simulink model "MDR_AA_TMD_Intercepteur"  (R2019b)
settings: Solver=ode4  StartTime=0.0  StopTime=Inf  FixedStep=0.01  RelTol=1e-3
values from neighbouring files (symbols this model uses):
  stdatm = [0 100 200 300 400 500 600 700 800 900 1000 1100 ... (4305 elements, 861x5)]    [stdatm.mat]
undefined symbols (not defined in the file or in its folder): Aero_Struct_CM, Aero_TMD, e0_0, e1_0, e2_0, e3_0, magnitude, Masse_Inertie_TMD, pow, Propu_TMD, Simu_TMD, Vm_0, xme_0
libraries: simulink x17
(part 2 of 4)

== system MDR_AA_TMD_Intercepteur/Intercepteur_TMD/Forces-Moments/Propulsion de l'exemple TMD ==
  <PS> : Inport
  Concaténation des deux phases de poussée : Subsystem
  Propulsion Booster : Subsystem  mask(Propulsion à poudre v1.0){Retard_Propu=Propu_TMD.Boost.Retard, t_b=Propu_TMD.Boost.Duree, Booster_Isp=Propu_TMD.Boost.ISP, Booster_Masse=Propu_TMD.Boost.Masse, Booster_Rapport=Propu_TMD.Boost.Profil, Diametre_tuy=Propu_TMD.Boost.D_Tuy, g0=9.80665}
      mask prompts: Retard_Propu "Retard Propulsion / T0 simu (s)"; t_b "Durée propulsion (s)"; Booster_Isp "Isp (s)"; Booster_Masse "Masse de poudre (kg)"; Booster_Rapport "Rapport de profil poussée (0->1)"; Diametre_tuy "Diamètre de la tuyere (m)"; g0 "Gravité au niveau du sol (m/s²)"
      mask help:
      | Modèle de propulseur à poudre.
      |
      | ENTREES
      | Pression_statique: Pression statique en Pa
      |
      | SORTIES
      | Force_poussee : Force de poussée axiale (en Newton)
      | débit_propu : Débit de combustible en kg.s^(-1)
      |
      | PARAMETRES
      | Retard Propulsion / T0 simu: délais entre le début de la simulation et l'allumage du propulseur
      | Durée propulsion: durée de la phase de propulsion (en s)
      | Isp: impulsion spécifique (en s)
      | Masse de poudre: Masse de propergol (en kg)
      | Rapport du profil de poussee (0->1): Allure du profil de poussée
      mask Help: eval('OpenHelp(''A3_NG.mdl'', ''Help\html\A3_NG_Model_Propu_Poudre_v10.html'')');
  Propulsion Croisiere : Subsystem  mask(Propulsion à poudre v1.0){Retard_Propu=Propu_TMD.Croisiere.Retard, t_b=Propu_TMD.Croisiere.Duree, Booster_Isp=Propu_TMD.Croisiere.ISP, Booster_Masse=Propu_TMD.Croisiere.Masse, Booster_Rapport=Propu_TMD.Croisiere.Profil, Diametre_tuy=Propu_TMD.Croisiere.D_Tuy, g0=9.80665}
      mask prompts: Retard_Propu "Retard Propulsion / T0 simu (s)"; t_b "Durée propulsion (s)"; Booster_Isp "Isp (s)"; Booster_Masse "Masse de poudre (kg)"; Booster_Rapport "Rapport de profil poussée (0->1)"; Diametre_tuy "Diamètre de la tuyere (m)"; g0 "Gravité au niveau du sol (m/s²)"
      mask help:
      | Modèle de propulseur à poudre.
      |
      | ENTREES
      | Pression_statique: Pression statique en Pa
      |
      | SORTIES
      | Force_poussee : Force de poussée axiale (en Newton)
      | débit_propu : Débit de combustible en kg.s^(-1)
      |
      | PARAMETRES
      | Retard Propulsion / T0 simu: délais entre le début de la simulation et l'allumage du propulseur
      | Durée propulsion: durée de la phase de propulsion (en s)
      | Isp: impulsion spécifique (en s)
      | Masse de poudre: Masse de propergol (en kg)
      | Rapport du profil de poussee (0->1): Allure du profil de poussée
      mask Help: eval('OpenHelp(''A3_NG.mdl'', ''Help\html\A3_NG_Model_Propu_Poudre_v10.html'')');
  Fpropu : Outport
  debit_carburant : Outport  Port=2
  wires:
  Concaténation des deux phases de poussée/2(debit_carburant) -> debit_carburant/1
  Propulsion Croisiere/2(debit_propu) -> Concaténation des deux phases de poussée/4(Debit_Croisiere)
  Propulsion Booster/1(Force_poussee) -> Concaténation des deux phases de poussée/1(Poussee_Boost)
  Propulsion Booster/2(debit_propu) -> Concaténation des deux phases de poussée/2(Poussee_Croisiere)
  Concaténation des deux phases de poussée/1(Fpropu) -> Fpropu/1
  <PS>/1 -> Propulsion Croisiere/1(Pression_statique), Propulsion Booster/1(Pression_statique)
  Propulsion Croisiere/1(Force_poussee) -> Concaténation des deux phases de poussée/3(Debit_Boost)

== system MDR_AA_TMD_Intercepteur/Modèle de terre/Modèle de terre WGS-84/Computation of Earth curvature radius (WGS-84) ==
  note: Computation of Earth curvature radius (WGS-84)
  Latitude : Inport
  1st Earth excentricity : Constant  Value=e
  Earth equatorial radius : Constant  Value=a
  Mux : Mux  Inputs=2
  Mux1 : Mux  Inputs=3
  Mux2 : Mux  Inputs=2
  Re = sqrt( Rmeridian * Rnormal ) : Fcn  Expr=sqrt(u(1)*u(2))
  "Rmeridian  = a ( 1 - e² ) / w^3 " : Fcn  Tag=Rmeridian  Expr=u(1)*(1-u(2)^2)/u(3)^3
  Rnormal = a / w : Fcn  Expr=u[1]/u[3]
  "w = sqrt ( 1 - e² sin² ( lat ) ) " : Fcn  Expr=sqrt(1-u(1)^2*sin(u(2))^2)
  Rmeridian : Outport  VectorParamsAs1DForOutWhenUnconnected=off
  Rnormal : Outport  Port=2  VectorParamsAs1DForOutWhenUnconnected=off
  Re : Outport  Port=3  VectorParamsAs1DForOutWhenUnconnected=off
  wires:
  "Rmeridian  = a ( 1 - e² ) / w^3 "/1 -> Rmeridian/1, Mux2/1
  Rnormal = a / w/1 -> Rnormal/1, Mux2/2
  Mux1/1 -> "Rmeridian  = a ( 1 - e² ) / w^3 "/1, Rnormal = a / w/1
  Earth equatorial radius/1 -> Mux1/1
  1st Earth excentricity/1 -> Mux/1, Mux1/2
  Latitude/1 -> Mux/2
  Re = sqrt( Rmeridian * Rnormal )/1 -> Re/1
  "w = sqrt ( 1 - e² sin² ( lat ) ) "/1 -> Mux1/3
  Mux/1 -> "w = sqrt ( 1 - e² sin² ( lat ) ) "/1
  Mux2/1 -> Re = sqrt( Rmeridian * Rnormal )/1

== system MDR_AA_TMD_Intercepteur/Modèle de terre/Modèle de terre WGS-84/Computation of the local gravity ==
  note: Computation of local gravity (WGS-84)
  Latitude : Inport
  Altitude : Inport  Port=2
  1st Earth excentricity : Constant  Value=e
  Earth equatorial radius : Constant  Value=a
  Ellipsoidal flattening : Constant  Value=f
  Gravity formula constant 1 : Constant  Value=k
  Gravity formula constant 2 : Constant  Value=m
  Mux : Mux  Inputs=6
  Mux1 : Mux
  Mux2 : Mux  Inputs=2
  Theoretical equatorial gravity : Constant  Value=ge
  g=ge*(1+k sin(lat)²)/w : Fcn  Expr=u(1)*(1+u(2)*sin(u(4))^2)/u(3)
  gh = g ( 1 - 2/a ( 1 + f + m - 2 f sin(lat)²) h + 3/a² h²) : Fcn  Expr=u[1]*(1-2/u[2]*(1+u[3]+u[4]-2*u[3]*sin(u[5])^2)*u[6]+3/u[2]^2*u[6]^2)
  "w = sqrt ( 1 - e² sin² ( lat ) ) " : Fcn  Expr=sqrt(1-u(1)^2*sin(u(2))^2)
  Gravity : Outport  VectorParamsAs1DForOutWhenUnconnected=off
  wires:
  Altitude/1 -> Mux/6
  Gravity formula constant 2/1 -> Mux/4
  Ellipsoidal flattening/1 -> Mux/3
  Earth equatorial radius/1 -> Mux/2
  g=ge*(1+k sin(lat)²)/w/1 -> Mux/1
  "w = sqrt ( 1 - e² sin² ( lat ) ) "/1 -> Mux1/3
  Mux2/1 -> "w = sqrt ( 1 - e² sin² ( lat ) ) "/1
  Latitude/1 -> Mux/5, Mux1/4, Mux2/2
  1st Earth excentricity/1 -> Mux2/1
  Mux/1 -> gh = g ( 1 - 2/a ( 1 + f + m - 2 f sin(lat)²) h + 3/a² h²)/1
  gh = g ( 1 - 2/a ( 1 + f + m - 2 f sin(lat)²) h + 3/a² h²)/1 -> Gravity/1
  Theoretical equatorial gravity/1 -> Mux1/1
  Gravity formula constant 1/1 -> Mux1/2
  Mux1/1 -> g=ge*(1+k sin(lat)²)/w/1

== system MDR_AA_TMD_Intercepteur/Modèle de terre/xyz_NED2LLA/ECEF2LLA ==
  ECEF : Inport
  Calcul de h : Subsystem
  Calcul de la latitude : Subsystem
  Calcul de la longitude : Subsystem
  Calcul de r : Subsystem
  Vector Concatenate1 : Concatenate  NumInputs=3
  LLA : Outport  VectorParamsAs1DForOutWhenUnconnected=off
  wires:
  ECEF/1 -> Calcul de r/1(xyz_ECEF), Calcul de h/3(xyz_ECEF), Calcul de la longitude/1(xyz_ECEF), Calcul de la latitude/1(xyz_ECEF)
  Calcul de h/1(h) -> Vector Concatenate1/3
  Vector Concatenate1/1 -> LLA/1
  Calcul de r/1(r) -> Calcul de la latitude/2(r), Calcul de h/2(r)
  Calcul de la longitude/1(Lambda) -> Vector Concatenate1/2
  Calcul de la latitude/1(Phi) -> Calcul de h/1(phi), Vector Concatenate1/1

== system MDR_AA_TMD_Intercepteur/Modèle de terre/xyz_NED2LLA/xyz_ENU2ECEF ==
  xyz_ENU : Inport
  Add : Sum
  Gain2 : Gain  Gain=[1;1;-1]
  Matrice de passage du repère NED au repère ECEF : Subsystem
  Product : Product  Multiplication=Matrix(*)
  Reshape : Reshape  OutputDimensionality=Column vector (2-D)
  Selector3 : Selector  InputPortWidth=3  IndexOptions=Index vector (dialog)  Indices=[2 1 3]  OutputSizes=1
  XYZ0 : Subsystem
  ECEF : Outport  VectorParamsAs1DForOutWhenUnconnected=off
  wires:
  xyz_ENU/1 -> Selector3/1
  Matrice de passage du repère NED au repère ECEF/1(M_NED2ECEF) -> Product/1
  XYZ0/1(XYZ0) -> Add/1
  Product/1 -> Add/2
  Add/1 -> ECEF/1
  Reshape/1 -> Product/2
  Gain2/1 -> Reshape/1
  Selector3/1 -> Gain2/1

== system MDR_AA_TMD_Intercepteur/Cible/Cible Cinématique v1.1/Actionneur Simulight/Retard Angle ==
  Angle_t_1 : Inport
  Angle_C : Inport  Port=2
  Tau : Inport  Port=3
  Constant1 : Constant
  Divide : Product  Inputs=*/
  Divide1 : Product  Inputs=**
  Gain : Gain  Gain=-1
  Gestion division par 0 : Subsystem
  Math Function : Math  SaturateOnIntegerOverflow=on
  Memory2 : Memory
  Ramp : simulink/Sources/Ramp  slope=1  start=0  InitialOutput=0
  Sum : Sum  Inputs=|-+
  Sum1 : Sum
  Sum2 : Sum  Inputs=-+
  Sum3 : Sum  Inputs=|+-
  Angle_R : Outport  VectorParamsAs1DForOutWhenUnconnected=off
  wires:
  Gestion division par 0/1(Non_zero) -> Divide/2
  Tau/1 -> Gestion division par 0/1(Zero_Possible)
  Angle_C/1 -> Sum2/2
  Divide1/1 -> Sum1/2
  Sum1/1 -> Angle_R/1
  Constant1/1 -> Sum/2
  Sum/1 -> Divide1/2
  Sum2/1 -> Divide1/1
  Math Function/1 -> Sum/1
  Gain/1 -> Divide/1
  Divide/1 -> Math Function/1
  Angle_t_1/1 -> Sum1/1, Sum2/1
  Ramp/1 -> Memory2/1, Sum3/1
  Memory2/1 -> Sum3/2
  Sum3/1 -> Gain/1

== system MDR_AA_TMD_Intercepteur/Cible/Cible Cinématique v1.1/Actionneur Simulight1/Retard Angle ==
  Angle_t_1 : Inport
  Angle_C : Inport  Port=2
  Tau : Inport  Port=3
  Constant1 : Constant
  Divide : Product  Inputs=*/
  Divide1 : Product  Inputs=**
  Gain : Gain  Gain=-1
  Gestion division par 0 : Subsystem
  Math Function : Math  SaturateOnIntegerOverflow=on
  Memory2 : Memory
  Ramp : simulink/Sources/Ramp  slope=1  start=0  InitialOutput=0
  Sum : Sum  Inputs=|-+
  Sum1 : Sum
  Sum2 : Sum  Inputs=-+
  Sum3 : Sum  Inputs=|+-
  Angle_R : Outport  VectorParamsAs1DForOutWhenUnconnected=off
  wires:
  Gestion division par 0/1(Non_zero) -> Divide/2
  Tau/1 -> Gestion division par 0/1(Zero_Possible)
  Angle_C/1 -> Sum2/2
  Divide1/1 -> Sum1/2
  Sum1/1 -> Angle_R/1
  Constant1/1 -> Sum/2
  Sum/1 -> Divide1/2
  Sum2/1 -> Divide1/1
  Math Function/1 -> Sum/1
  Gain/1 -> Divide/1
  Divide/1 -> Math Function/1
  Angle_t_1/1 -> Sum1/1, Sum2/1
  Ramp/1 -> Memory2/1, Sum3/1
  Memory2/1 -> Sum3/2
  Sum3/1 -> Gain/1

== system MDR_AA_TMD_Intercepteur/Cible/Cible Cinématique v1.1/Aero/Norme ==
  V : Inport
  Dot Product : DotProduct  InputSameDT=on  OutDataTypeStr=Inherit: Inherit via internal rule
  Sqrt : Math  Operator=sqrt  SaturateOnIntegerOverflow=on
  ||V|| : Outport  VectorParamsAs1DForOutWhenUnconnected=off
  wires:
  Sqrt/1 -> ||V||/1
  V/1 -> Dot Product/2, Dot Product/1
  Dot Product/1 -> Sqrt/1

== system MDR_AA_TMD_Intercepteur/Cible/Cible Cinématique v1.1/Aero/q\ ==
  ||V|| : Inport
  Rho : Inport  Port=2
  Gain : Gain  Gain=0.5
  Gain1 : Gain  Gain=(Lref^2*pi)/4
  Math Function : Math  Operator=magnitude^2  SaturateOnIntegerOverflow=on
  Product2 : Product  RndMeth=Zero
  rsv2 : Outport  VectorParamsAs1DForOutWhenUnconnected=off
  wires:
  Gain/1 -> Product2/1
  ||V||/1 -> Math Function/1
  Rho/1 -> Gain/1
  Product2/1 -> Gain1/1
  Math Function/1 -> Product2/2
  Gain1/1 -> rsv2/1

== system MDR_AA_TMD_Intercepteur/Cible/Cible Cinématique v1.1/Cinématique 6ddl Simulight avec pilotage en force/Calcul de la vitesse engin dans le repère inertiel ==
  Vb : Inport
  e0e1e2e3 : Inport  Port=2
  Math Function : Math  Operator=transpose  SaturateOnIntegerOverflow=on
  Product : Product  Multiplication=Matrix(*)  SaturateOnIntegerOverflow=on  InputSameDT=on  OutDataTypeStr=Inherit: Same as first input
  Quaternion2DCM : Subsystem  mask(Quaternion2DCM){}
      mask help:
      | Calcul la matrice de passage DCM (Direct Cosine Matrix) à partir du quaternion q.
      |
      | Si q = q0+ q1 i + q2 j + q3 k alors
      |
      | DCM = [
      | 1-2q2^2-2q3^2	2q1q2-2q0q3	2q1q3+2q0q2
      | 2q1q2+2q0q3	1-2q1^2-2q3^2	2q2q3-2q0q1
      | 2q1q3-2q0q2	2q2q3+2q0q1	1-2q1^2-2q2^2
      | ]
      mask Help: eval('OpenHelp(''A3_NG.mdl'', ''Help\html\A3_NG_Model_Quaternion2DCM.html'')');
  Ve : Outport  VectorParamsAs1DForOutWhenUnconnected=off
  wires:
  Vb/1 -> Product/2
  Math Function/1 -> Product/1
  e0e1e2e3/1 -> Quaternion2DCM/1(Quaternion)
  Quaternion2DCM/1(DCM) -> Math Function/1
  Product/1 -> Ve/1

== system MDR_AA_TMD_Intercepteur/Cible/Cible Cinématique v1.1/Cinématique 6ddl Simulight avec pilotage en force/Calcul des pqr ==
  Ab : Inport
  Vb : Inport  Port=2
  AlphaR : Inport  Port=3
  BetaR : Inport  Port=4
  pqr_force : Inport  Port=5
  Add : Sum  Inputs=+++
  pqr_a : Subsystem
  pqr_b : Subsystem
  pqr : Outport  VectorParamsAs1DForOutWhenUnconnected=off
  wires:
  AlphaR/1 -> pqr_a/1(AlphaR)
  BetaR/1 -> pqr_a/2(BetaR)
  pqr_a/1(pqr_a) -> Add/2
  pqr_b/1(pqr_b) -> Add/1
  Ab/1 -> pqr_b/1(Ab)
  Vb/1 -> pqr_b/2(Vb)
  Add/1 -> pqr/1
  pqr_force/1 -> Add/3

== system MDR_AA_TMD_Intercepteur/Cible/Cible Cinématique v1.1/Cinématique 6ddl Simulight avec pilotage en force/Equations des forces ==
  g : Inport
  Faero : Inport  Port=2
  Masse : Inport  Port=3
  pqr : Inport  Port=4
  Divide : Product  Inputs=*/
  Gestion de sortie de rampe : Subsystem
  "Sous contrainte de la rampe, effort uniquement sur l'axe longitudinal" : Subsystem
  Switch : Switch  Criteria=u2 ~= 0
  U^V : Subsystem  mask(Produit Vectoriel){}
      mask help: Calcul le produit vectoriel de deux vecteur 3x1.
      mask Help: eval('OpenHelp(''A3_NG.mdl'', ''Help\html\A3_NG_Model_ProdVect.html'')');
      mask Display: disp('Produit\nVectoriel')
  m3 : Constant  Value=Vb0
  sum : Sum  Inputs=|++  SaturateOnIntegerOverflow=on  InputSameDT=on  OutDataTypeStr=Inherit: Same as first input
  sum1 : Sum  SaturateOnIntegerOverflow=on  InputSameDT=on  OutDataTypeStr=Inherit: Same as first input
  ub vb wb : Integrator  InitialConditionSource=external  InitialCondition=Vm_0
  Vb : Outport  VectorParamsAs1DForOutWhenUnconnected=off
  Ab : Outport  Port=2  VectorParamsAs1DForOutWhenUnconnected=off
  wires:
  U^V/1(c(1) c(2) c(3)) -> sum/2
  m3/1 -> ub vb wb/2
  sum/1 -> ub vb wb/1
  ub vb wb/1 -> Vb/1, U^V/1(a(1) a(2) a(3))
  pqr/1 -> U^V/2(b(1) b(2) b(3))
  Faero/1 -> Divide/1
  Masse/1 -> Divide/2
  Divide/1 -> sum1/2, Gestion de sortie de rampe/1(Fm)
  g/1 -> sum1/1
  sum1/1 -> "Sous contrainte de la rampe, effort uniquement sur l'axe longitudinal"/1(F), Switch/1
  Switch/1 -> Ab/1, sum/1
  Gestion de sortie de rampe/1(Sortie_Rampe) -> Switch/2
  "Sous contrainte de la rampe, effort uniquement sur l'axe longitudinal"/1(Fx) -> Switch/3

== system MDR_AA_TMD_Intercepteur/Cible/Cible Cinématique v1.1/Cinématique 6ddl Simulight avec pilotage en force/Intégration de la vitesse dans le repère inertiel ==
  Ve : Inport
  m2 : Constant  Value=Xe0
  xe ye ze : Integrator  InitialConditionSource=external  InitialCondition=xme_0
  Xe : Outport  VectorParamsAs1DForOutWhenUnconnected=off
  wires:
  m2/1 -> xe ye ze/2
  Ve/1 -> xe ye ze/1
  xe ye ze/1 -> Xe/1

== system MDR_AA_TMD_Intercepteur/Cible/Cible Cinématique v1.1/Cinématique 6ddl Simulight avec pilotage en force/Pesanteur ==
  Euler : Inport
  g : Inport  Port=2
  Gain : Gain  Gain=[0;0;1]
  Inert2Miss : Subsystem  mask(Inert2Miss){}
      mask help: Calcul les composantes d'un vecteur du repère inertiel dans le repère missile.
      mask Help: eval('OpenHelp(''A3_NG.mdl'', ''Help\html\A3_NG_Model_Inert2Miss.html'')');
  g_miss : Outport  VectorParamsAs1DForOutWhenUnconnected=off
  wires:
  Euler/1 -> Inert2Miss/1(Euler)
  g/1 -> Gain/1
  Gain/1 -> Inert2Miss/2(U)
  Inert2Miss/1(V) -> g_miss/1

== system MDR_AA_TMD_Intercepteur/Cible/Cible Cinématique v1.1/Cinématique 6ddl Simulight avec pilotage en force/Quaternion2Euler ==
  Quaternion : Inport  PortDimensions=[4 1]
  Fcn1 : Fcn  Expr=atan2( 2*(u(1)*u(2)+u(3)*u(4)),u(1)^2-u(2)^2-u(3)^2+u(4)^2 )
  Fcn3 : Fcn  Expr=atan2( 2*(u(2)*u(3)+u(1)*u(4)),u(1)^2+u(2)^2-u(3)^2-u(4)^2 )
  Fcn4 : Fcn  Expr=2*(u(1)*u(3)-u(2)*u(4))
  Fcn5 : Fcn  Expr=asin(u(1))
  Mux : Mux  Inputs=3
  Saturation : Saturate  UpperLimit=1  LowerLimit=-1
  Euler : Outport  VectorParamsAs1DForOutWhenUnconnected=off
  wires:
  Fcn5/1 -> Mux/2
  Saturation/1 -> Fcn5/1
  Fcn4/1 -> Saturation/1
  Quaternion/1 -> Fcn1/1, Fcn4/1, Fcn3/1
  Fcn3/1 -> Mux/3
  Mux/1 -> Euler/1
  Fcn1/1 -> Mux/1

== system MDR_AA_TMD_Intercepteur/Cible/Cible Cinématique v1.1/Cinématique 6ddl Simulight avec pilotage en force/pqr2Quaternion ==
  pqr : Inport
  Constant1 : Constant  Value=Euler_Init
  Divide : Product  Inputs=*/
  Euler2Quaternion : Subsystem  mask(Euler2Quaternion){}
      mask help:
      | Calcul du quaternion q à partir des angles d'Euler (phi,theta,psi)
      |
      | q = q0 + q1 i + q2 j + q3 k
      | avec :
      |
      | q0 = cos(0.5*psi)cos(0.5*theta)cos(0.5*phi) + sin(0.5*psi)sin(0.5*theta)sin(0.5*phi)
      | q1 =  sin(0.5*psi)cos(0.5*theta)cos(0.5*phi) - cos(0.5*psi)sin(0.5*theta)sin(0.5*phi)
      | q2 =  cos(0.5*psi)sin(0.5*theta)cos(0.5*phi) + sin(0.5*psi)cos(0.5*theta)sin(0.5*phi)
      | q3 =  cos(0.5*psi)cos(0.5*theta)sin(0.5*phi) - sin(0.5*psi)sin(0.5*theta)cos(0.5*phi)
      mask Help: eval('OpenHelp(''A3_NG.mdl'', ''Help\html\A3_NG_Model_Euler2Quaternion.html'')');
  Norme : Subsystem  mask(Norme){}
      mask help: Calcul la norme quadratique d'un vecteur.
      mask Help: eval('OpenHelp(''A3_NG.mdl'', ''Help\html\A3_NG_Model_Norme.html'')');
  deg2rad : Gain  Gain=pi/180
  e0 e1 e2 e3 : Integrator  InitialConditionSource=external  InitialCondition=[e0_0 e1_0 e2_0 e3_0]
  pqr to eidot : Subsystem
  Quaternion : Outport  VectorParamsAs1DForOutWhenUnconnected=off
  wires:
  deg2rad/1 -> Euler2Quaternion/1(Euler)
  pqr/1 -> pqr to eidot/1(pqr)
  Divide/1 -> Quaternion/1, pqr to eidot/2(e0e1e2e3)
  Norme/1(||V||) -> Divide/2
  e0 e1 e2 e3/1 -> Divide/1, Norme/1(V)
  Constant1/1 -> deg2rad/1
  pqr to eidot/1(eidot) -> e0 e1 e2 e3/1
  Euler2Quaternion/1(Quaternion) -> e0 e1 e2 e3/2

== system MDR_AA_TMD_Intercepteur/Cible/Cible Cinématique v1.1/Pilote 2 axes Simulight à partir de gradient/Alpha commandé - Plan de tangage ==
  GcoV : Inport
  Masse : Inport  Port=2
  Pression_dynamique : Inport  Port=3
  Compare To Zero : simulink/Logic and Bit Operations/Compare To Zero  relop===  OutDataTypeStr=boolean  ZeroCross=off
  Cza : Gain  Gain=Cza
  Divide1 : Product  Inputs=*/
  Memory : Memory
  Product : Product  RndMeth=Zero
  Switch : Switch  Criteria=u2 > Threshold
  Zero Offset : Subsystem  mask(Zero offset){tol=10^-6}
      mask prompts: tol "Tolerance"
      mask help: This block outputs a value equal to the tolerance specified in the block parameters if the input falls within a sphere with this tolerance as radius and center in the origin. Otherwise, the output equals the input.
      mask Help: eval('OpenHelp(''A3_Blockset.mdl'', ''..\Help\Toolbox\Tools\Zero_offset.html'')');
  Alphaco : Outport  PortDimensions=1  VectorParamsAs1DForOutWhenUnconnected=off
  wires:
  Cza/1 -> Compare To Zero/1, Zero Offset/1(In)
  Zero Offset/1(Out) -> Divide1/2
  Memory/1 -> Switch/1
  Product/1 -> Switch/3
  Divide1/1 -> Product/1
  Masse/1 -> Divide1/1
  GcoV/1 -> Product/2
  Compare To Zero/1 -> Switch/2
  Switch/1 -> Alphaco/1, Memory/1
  Pression_dynamique/1 -> Cza/1

== system MDR_AA_TMD_Intercepteur/Cible/Cible Cinématique v1.1/Pilote 2 axes Simulight à partir de gradient/Beta commandé - Plan de lacet ==
  GcoH : Inport
  Masse : Inport  Port=2
  Pression_dynamique : Inport  Port=3
  Compare To Zero : simulink/Logic and Bit Operations/Compare To Zero  relop===  OutDataTypeStr=boolean  ZeroCross=off
  Cyb : Gain  Gain=Cyb
  Divide1 : Product  Inputs=*/
  Memory : Memory
  Product : Product  RndMeth=Zero
  Switch : Switch  Criteria=u2 > Threshold
  Zero Offset : Subsystem  mask(Zero offset){tol=10^-6}
      mask prompts: tol "Tolerance"
      mask help: This block outputs a value equal to the tolerance specified in the block parameters if the input falls within a sphere with this tolerance as radius and center in the origin. Otherwise, the output equals the input.
      mask Help: eval('OpenHelp(''A3_Blockset.mdl'', ''..\Help\Toolbox\Tools\Zero_offset.html'')');
  Betaco : Outport  PortDimensions=1  VectorParamsAs1DForOutWhenUnconnected=off
  wires:
  Pression_dynamique/1 -> Cyb/1
  Switch/1 -> Memory/1, Betaco/1
  Compare To Zero/1 -> Switch/2
  GcoH/1 -> Product/2
  Masse/1 -> Divide1/1
  Divide1/1 -> Product/1
  Product/1 -> Switch/3
  Memory/1 -> Switch/1
  Zero Offset/1(Out) -> Divide1/2
  Cyb/1 -> Zero Offset/1(In), Compare To Zero/1

== system MDR_AA_TMD_Intercepteur/Cible/Cible Cinématique v1.1/Pilote 2 axes Simulight à partir de gradient/Norme ==
  V : Inport
  Dot Product : DotProduct  InputSameDT=on  OutDataTypeStr=Inherit: Inherit via internal rule
  Sqrt : Math  Operator=sqrt  SaturateOnIntegerOverflow=on
  ||V|| : Outport  VectorParamsAs1DForOutWhenUnconnected=off
  wires:
  Sqrt/1 -> ||V||/1
  V/1 -> Dot Product/2, Dot Product/1
  Dot Product/1 -> Sqrt/1

== system MDR_AA_TMD_Intercepteur/Cible/Cible Cinématique v1.1/Pilote 2 axes Simulight à partir de gradient/q\ ==
  ||V|| : Inport
  Rho : Inport  Port=2
  Gain : Gain  Gain=0.5
  Gain1 : Gain  Gain=(Lref^2*pi)/4
  Math Function : Math  Operator=magnitude^2  SaturateOnIntegerOverflow=on
  Product2 : Product  RndMeth=Zero
  rsv2 : Outport  VectorParamsAs1DForOutWhenUnconnected=off
  wires:
  Gain/1 -> Product2/1
  ||V||/1 -> Math Function/1
  Rho/1 -> Gain/1
  Product2/1 -> Gain1/1
  Math Function/1 -> Product2/2
  Gain1/1 -> rsv2/1

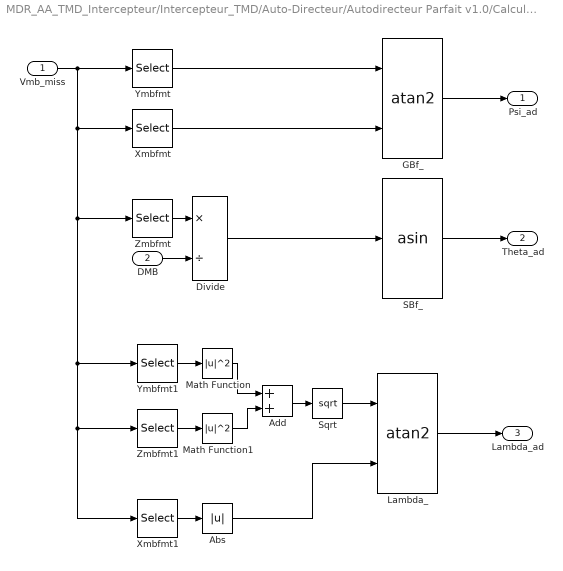
== system MDR_AA_TMD_Intercepteur/Intercepteur_TMD/Auto-Directeur/Autodirecteur Parfait v1.0/Calcul des angles site et gisement de la droite missile//but dans le repère missile ==
  Vmb_miss : Inport
  DMB : Inport  Port=2
  Abs : Abs
  Add : Sum
  Divide : Product  Inputs=*/
  GBf_ : Trigonometry  Operator=atan2
  Lambda_ : Trigonometry  Operator=atan2
  Math Function : Math  Operator=magnitude^2  SaturateOnIntegerOverflow=on
  Math Function1 : Math  Operator=magnitude^2  SaturateOnIntegerOverflow=on
  SBf_ : Trigonometry  Operator=asin
  Sqrt : Sqrt  SaturateOnIntegerOverflow=on
  Xmbfmt : Selector  InputPortWidth=3  IndexOptions=Index vector (dialog)  Indices=[1]  OutputSizes=1
  Xmbfmt1 : Selector  InputPortWidth=3  IndexOptions=Index vector (dialog)  Indices=[1]  OutputSizes=1
  Ymbfmt : Selector  InputPortWidth=3  IndexOptions=Index vector (dialog)  Indices=[2]  OutputSizes=1
  Ymbfmt1 : Selector  InputPortWidth=3  IndexOptions=Index vector (dialog)  Indices=[2]  OutputSizes=1
  Zmbfmt : Selector  InputPortWidth=3  IndexOptions=Index vector (dialog)  Indices=[3]  OutputSizes=1
  Zmbfmt1 : Selector  InputPortWidth=3  IndexOptions=Index vector (dialog)  Indices=[3]  OutputSizes=1
  Psi_ad : Outport  VectorParamsAs1DForOutWhenUnconnected=off
  Theta_ad : Outport  Port=2  VectorParamsAs1DForOutWhenUnconnected=off
  Lambda_ad : Outport  Port=3  VectorParamsAs1DForOutWhenUnconnected=off
  wires:
  DMB/1 -> Divide/2
  Divide/1 -> SBf_/1
  Zmbfmt/1 -> Divide/1
  SBf_/1 -> Theta_ad/1
  GBf_/1 -> Psi_ad/1
  Xmbfmt/1 -> GBf_/2
  Ymbfmt/1 -> GBf_/1
  Vmb_miss/1 -> Ymbfmt/1, Xmbfmt/1, Zmbfmt/1, Ymbfmt1/1, Zmbfmt1/1, Xmbfmt1/1
  Add/1 -> Sqrt/1
  Ymbfmt1/1 -> Math Function/1
  Math Function/1 -> Add/1
  Zmbfmt1/1 -> Math Function1/1
  Math Function1/1 -> Add/2
  Sqrt/1 -> Lambda_/1
  Xmbfmt1/1 -> Abs/1
  Abs/1 -> Lambda_/2
  Lambda_/1 -> Lambda_ad/1

== system MDR_AA_TMD_Intercepteur/Intercepteur_TMD/Auto-Directeur/Autodirecteur Parfait v1.0/Calcul des vitesses de défilements de la droite missile//but dans le repère missile ==
  Omega_miss : Inport
  Gain : Gain  Gain=-1
  omega ymt : Selector  InputPortWidth=3  IndexOptions=Index vector (dialog)  Indices=[2]  OutputSizes=1
  omega zmt : Selector  InputPortWidth=3  IndexOptions=Index vector (dialog)  Indices=[3]  OutputSizes=1
  wzad : Outport  VectorParamsAs1DForOutWhenUnconnected=off
  wyad : Outport  Port=2  VectorParamsAs1DForOutWhenUnconnected=off
  wires:
  omega zmt/1 -> wyad/1
  omega ymt/1 -> Gain/1
  Omega_miss/1 -> omega ymt/1, omega zmt/1
  Gain/1 -> wzad/1

== system MDR_AA_TMD_Intercepteur/Intercepteur_TMD/Auto-Directeur/Autodirecteur Parfait v1.0/Calcul du vecteur rotation instantané de la droite missile//but dans le repère inertiel ==
  Pos_Miss_inert : Inport
  Pos_Cible_inert : Inport  Port=2
  Vit_Miss_inert : Inport  Port=3
  Vit_Cible_inert : Inport  Port=4
  Add : Sum  Inputs=+-
  Add1 : Sum  Inputs=+-
  Divide : Product  Inputs=*/
  Math Function1 : Math  Operator=magnitude^2  SaturateOnIntegerOverflow=on
  Norme : Subsystem  mask(Norme){}
      mask help: Calcul la norme quadratique d'un vecteur.
      mask Help: eval('OpenHelp(''A3_NG.mdl'', ''Help\html\A3_NG_Model_Norme.html'')');
  U^V : Subsystem  mask(Produit Vectoriel){}
      mask help: Calcul le produit vectoriel de deux vecteur 3x1.
      mask Help: eval('OpenHelp(''A3_NG.mdl'', ''Help\html\A3_NG_Model_ProdVect.html'')');
      mask Display: disp('Produit\nVectoriel')
  Omega_inert : Outport  VectorParamsAs1DForOutWhenUnconnected=off
  wires:
  Divide/1 -> Omega_inert/1  "NPi"
  Norme/1(||V||) -> Math Function1/1
  Pos_Cible_inert/1 -> Add/1
  Pos_Miss_inert/1 -> Add/2
  Add/1 -> U^V/1(a(1) a(2) a(3)), Norme/1(V)  "dX"
  Vit_Miss_inert/1 -> Add1/2
  Vit_Cible_inert/1 -> Add1/1
  Add1/1 -> U^V/2(b(1) b(2) b(3))  "dV"
  U^V/1(c(1) c(2) c(3)) -> Divide/1
  Math Function1/1 -> Divide/2

== system MDR_AA_TMD_Intercepteur/Intercepteur_TMD/Auto-Directeur/Autodirecteur Parfait v1.0/Changement de repère inertiel -> miss ==
  Euler : Inport
  Omega_inert : Inport  Port=2
  Vmb_inert : Inport  Port=3
  Inert2Miss1 : Subsystem  mask(Inert2Miss){}
      mask help: Calcul les composantes d'un vecteur du repère inertiel dans le repère missile.
      mask Help: eval('OpenHelp(''A3_NG.mdl'', ''Help\html\A3_NG_Model_Inert2Miss.html'')');
  Matrix Concatenate : Concatenate  Mode=Multidimensional array  ConcatenateDimension=2
  Selector : Selector  NumberOfDimensions=2  InputPortWidth=[3 2]  IndexOptions=Select all,Index vector (dialog)  Indices=[1],1  OutputSizes=1,1
  Selector1 : Selector  NumberOfDimensions=2  InputPortWidth=[3 2]  IndexOptions=Select all,Index vector (dialog)  Indices=[1 3],2  OutputSizes=1,1
  Omega_miss : Outport  VectorParamsAs1DForOutWhenUnconnected=off
  Vmb_miss : Outport  Port=2  VectorParamsAs1DForOutWhenUnconnected=off
  wires:
  Euler/1 -> Inert2Miss1/1(Euler)
  Omega_inert/1 -> Matrix Concatenate/1
  Vmb_inert/1 -> Matrix Concatenate/2
  Matrix Concatenate/1 -> Inert2Miss1/2(U)
  Inert2Miss1/1(V) -> Selector/1, Selector1/1
  Selector/1 -> Omega_miss/1
  Selector1/1 -> Vmb_miss/1

== system MDR_AA_TMD_Intercepteur/Intercepteur_TMD/Auto-Directeur/Autodirecteur Parfait v1.0/Site et Gisement de la droite missile//but dans le repère inertiel ==
  Pos_Cible_inert : Inport
  Pos_Miss_inert : Inport  Port=2
  Add : Sum  Inputs=+-
  Norme : Subsystem  mask(Norme){}
      mask help: Calcul la norme quadratique d'un vecteur.
      mask Help: eval('OpenHelp(''A3_NG.mdl'', ''Help\html\A3_NG_Model_Norme.html'')');
  Vector Concatenate : Concatenate  NumInputs=3
  Xb : Selector  InputPortWidth=3  IndexOptions=Index vector (dialog)  Indices=[1]  OutputSizes=1
  Xb-Xm : Sum  Inputs=+-
  Xb-Xm1 : Sum  Inputs=+-
  Xm : Selector  InputPortWidth=3  IndexOptions=Index vector (dialog)  Indices=[1]  OutputSizes=1
  Yb : Selector  InputPortWidth=3  IndexOptions=Index vector (dialog)  Indices=[2]  OutputSizes=1
  Yb-Ym : Sum  Inputs=+-
  Ym : Selector  InputPortWidth=3  IndexOptions=Index vector (dialog)  Indices=[2]  OutputSizes=1
  Zb : Selector  InputPortWidth=3  IndexOptions=Index vector (dialog)  Indices=[3]  OutputSizes=1
  Zm : Selector  InputPortWidth=3  IndexOptions=Index vector (dialog)  Indices=[3]  OutputSizes=1
  Vmb_inert : Outport  VectorParamsAs1DForOutWhenUnconnected=off
  DMB : Outport  Port=2  VectorParamsAs1DForOutWhenUnconnected=off
  wires:
  Yb/1 -> Yb-Ym/1
  Ym/1 -> Yb-Ym/2
  Xb/1 -> Xb-Xm/1
  Xm/1 -> Xb-Xm/2
  Zb/1 -> Xb-Xm1/1
  Zm/1 -> Xb-Xm1/2
  Pos_Cible_inert/1 -> Zb/1, Add/1, Yb/1, Xb/1
  Pos_Miss_inert/1 -> Zm/1, Add/2, Ym/1, Xm/1
  Norme/1(||V||) -> DMB/1
  Add/1 -> Norme/1(V)
  Vector Concatenate/1 -> Vmb_inert/1
  Xb-Xm/1 -> Vector Concatenate/1
  Yb-Ym/1 -> Vector Concatenate/2
  Xb-Xm1/1 -> Vector Concatenate/3

== system MDR_AA_TMD_Intercepteur/Intercepteur_TMD/Bloc Cinématique/Cinématique 6ddl Simulight avec pilotage en force/Calcul de la vitesse engin dans le repère inertiel ==
  Vb : Inport
  e0e1e2e3 : Inport  Port=2
  Math Function : Math  Operator=transpose  SaturateOnIntegerOverflow=on
  Product : Product  Multiplication=Matrix(*)  SaturateOnIntegerOverflow=on  InputSameDT=on  OutDataTypeStr=Inherit: Same as first input
  Quaternion2DCM : Subsystem  mask(Quaternion2DCM){}
      mask help:
      | Calcul la matrice de passage DCM (Direct Cosine Matrix) à partir du quaternion q.
      |
      | Si q = q0+ q1 i + q2 j + q3 k alors
      |
      | DCM = [
      | 1-2q2^2-2q3^2	2q1q2-2q0q3	2q1q3+2q0q2
      | 2q1q2+2q0q3	1-2q1^2-2q3^2	2q2q3-2q0q1
      | 2q1q3-2q0q2	2q2q3+2q0q1	1-2q1^2-2q2^2
      | ]
      mask Help: eval('OpenHelp(''A3_NG.mdl'', ''Help\html\A3_NG_Model_Quaternion2DCM.html'')');
  Ve : Outport  VectorParamsAs1DForOutWhenUnconnected=off
  wires:
  Vb/1 -> Product/2
  Math Function/1 -> Product/1
  e0e1e2e3/1 -> Quaternion2DCM/1(Quaternion)
  Quaternion2DCM/1(DCM) -> Math Function/1
  Product/1 -> Ve/1

== system MDR_AA_TMD_Intercepteur/Intercepteur_TMD/Bloc Cinématique/Cinématique 6ddl Simulight avec pilotage en force/Calcul des pqr ==
  Ab : Inport
  Vb : Inport  Port=2
  AlphaR : Inport  Port=3
  BetaR : Inport  Port=4
  pqr_force : Inport  Port=5
  Add : Sum  Inputs=+++
  pqr_a : Subsystem
  pqr_b : Subsystem
  pqr : Outport  VectorParamsAs1DForOutWhenUnconnected=off
  wires:
  AlphaR/1 -> pqr_a/1(AlphaR)
  BetaR/1 -> pqr_a/2(BetaR)
  pqr_a/1(pqr_a) -> Add/2
  pqr_b/1(pqr_b) -> Add/1
  Ab/1 -> pqr_b/1(Ab)
  Vb/1 -> pqr_b/2(Vb)
  Add/1 -> pqr/1
  pqr_force/1 -> Add/3

== system MDR_AA_TMD_Intercepteur/Intercepteur_TMD/Bloc Cinématique/Cinématique 6ddl Simulight avec pilotage en force/Equations des forces ==
  g : Inport
  Faero : Inport  Port=2
  Masse : Inport  Port=3
  pqr : Inport  Port=4
  Divide : Product  Inputs=*/
  Gestion de sortie de rampe : Subsystem
  "Sous contrainte de la rampe, effort uniquement sur l'axe longitudinal" : Subsystem
  Switch : Switch  Criteria=u2 ~= 0
  U^V : Subsystem  mask(Produit Vectoriel){}
      mask help: Calcul le produit vectoriel de deux vecteur 3x1.
      mask Help: eval('OpenHelp(''A3_NG.mdl'', ''Help\html\A3_NG_Model_ProdVect.html'')');
      mask Display: disp('Produit\nVectoriel')
  m3 : Constant  Value=Vb0
  sum : Sum  Inputs=|++  SaturateOnIntegerOverflow=on  InputSameDT=on  OutDataTypeStr=Inherit: Same as first input
  sum1 : Sum  SaturateOnIntegerOverflow=on  InputSameDT=on  OutDataTypeStr=Inherit: Same as first input
  ub vb wb : Integrator  InitialConditionSource=external  InitialCondition=Vm_0
  Vb : Outport  VectorParamsAs1DForOutWhenUnconnected=off
  Ab : Outport  Port=2  VectorParamsAs1DForOutWhenUnconnected=off
  wires:
  U^V/1(c(1) c(2) c(3)) -> sum/2
  m3/1 -> ub vb wb/2
  sum/1 -> ub vb wb/1
  ub vb wb/1 -> Vb/1, U^V/1(a(1) a(2) a(3))
  pqr/1 -> U^V/2(b(1) b(2) b(3))
  Faero/1 -> Divide/1
  Masse/1 -> Divide/2
  Divide/1 -> sum1/2, Gestion de sortie de rampe/1(Fm)
  g/1 -> sum1/1
  sum1/1 -> "Sous contrainte de la rampe, effort uniquement sur l'axe longitudinal"/1(F), Switch/1
  Switch/1 -> Ab/1, sum/1
  Gestion de sortie de rampe/1(Sortie_Rampe) -> Switch/2
  "Sous contrainte de la rampe, effort uniquement sur l'axe longitudinal"/1(Fx) -> Switch/3

== system MDR_AA_TMD_Intercepteur/Intercepteur_TMD/Bloc Cinématique/Cinématique 6ddl Simulight avec pilotage en force/Intégration de la vitesse dans le repère inertiel ==
  Ve : Inport
  m2 : Constant  Value=Xe0
  xe ye ze : Integrator  InitialConditionSource=external  InitialCondition=xme_0
  Xe : Outport  VectorParamsAs1DForOutWhenUnconnected=off
  wires:
  m2/1 -> xe ye ze/2
  Ve/1 -> xe ye ze/1
  xe ye ze/1 -> Xe/1

== system MDR_AA_TMD_Intercepteur/Intercepteur_TMD/Bloc Cinématique/Cinématique 6ddl Simulight avec pilotage en force/Pesanteur ==
  Euler : Inport
  g : Inport  Port=2
  Gain : Gain  Gain=[0;0;1]
  Inert2Miss : Subsystem  mask(Inert2Miss){}
      mask help: Calcul les composantes d'un vecteur du repère inertiel dans le repère missile.
      mask Help: eval('OpenHelp(''A3_NG.mdl'', ''Help\html\A3_NG_Model_Inert2Miss.html'')');
  g_miss : Outport  VectorParamsAs1DForOutWhenUnconnected=off
  wires:
  Euler/1 -> Inert2Miss/1(Euler)
  g/1 -> Gain/1
  Gain/1 -> Inert2Miss/2(U)
  Inert2Miss/1(V) -> g_miss/1

== system MDR_AA_TMD_Intercepteur/Intercepteur_TMD/Bloc Cinématique/Cinématique 6ddl Simulight avec pilotage en force/Quaternion2Euler ==
  Quaternion : Inport  PortDimensions=[4 1]
  Fcn1 : Fcn  Expr=atan2( 2*(u(1)*u(2)+u(3)*u(4)),u(1)^2-u(2)^2-u(3)^2+u(4)^2 )
  Fcn3 : Fcn  Expr=atan2( 2*(u(2)*u(3)+u(1)*u(4)),u(1)^2+u(2)^2-u(3)^2-u(4)^2 )
  Fcn4 : Fcn  Expr=2*(u(1)*u(3)-u(2)*u(4))
  Fcn5 : Fcn  Expr=asin(u(1))
  Mux : Mux  Inputs=3
  Saturation : Saturate  UpperLimit=1  LowerLimit=-1
  Euler : Outport  VectorParamsAs1DForOutWhenUnconnected=off
  wires:
  Fcn5/1 -> Mux/2
  Saturation/1 -> Fcn5/1
  Fcn4/1 -> Saturation/1
  Quaternion/1 -> Fcn1/1, Fcn4/1, Fcn3/1
  Fcn3/1 -> Mux/3
  Mux/1 -> Euler/1
  Fcn1/1 -> Mux/1

== system MDR_AA_TMD_Intercepteur/Intercepteur_TMD/Bloc Cinématique/Cinématique 6ddl Simulight avec pilotage en force/pqr2Quaternion ==
  pqr : Inport
  Constant1 : Constant  Value=Euler_Init
  Divide : Product  Inputs=*/
  Euler2Quaternion : Subsystem  mask(Euler2Quaternion){}
      mask help:
      | Calcul du quaternion q à partir des angles d'Euler (phi,theta,psi)
      |
      | q = q0 + q1 i + q2 j + q3 k
      | avec :
      |
      | q0 = cos(0.5*psi)cos(0.5*theta)cos(0.5*phi) + sin(0.5*psi)sin(0.5*theta)sin(0.5*phi)
      | q1 =  sin(0.5*psi)cos(0.5*theta)cos(0.5*phi) - cos(0.5*psi)sin(0.5*theta)sin(0.5*phi)
      | q2 =  cos(0.5*psi)sin(0.5*theta)cos(0.5*phi) + sin(0.5*psi)cos(0.5*theta)sin(0.5*phi)
      | q3 =  cos(0.5*psi)cos(0.5*theta)sin(0.5*phi) - sin(0.5*psi)sin(0.5*theta)cos(0.5*phi)
      mask Help: eval('OpenHelp(''A3_NG.mdl'', ''Help\html\A3_NG_Model_Euler2Quaternion.html'')');
  Norme : Subsystem  mask(Norme){}
      mask help: Calcul la norme quadratique d'un vecteur.
      mask Help: eval('OpenHelp(''A3_NG.mdl'', ''Help\html\A3_NG_Model_Norme.html'')');
  deg2rad : Gain  Gain=pi/180
  e0 e1 e2 e3 : Integrator  InitialConditionSource=external  InitialCondition=[e0_0 e1_0 e2_0 e3_0]
  pqr to eidot : Subsystem
  Quaternion : Outport  VectorParamsAs1DForOutWhenUnconnected=off
  wires:
  deg2rad/1 -> Euler2Quaternion/1(Euler)
  pqr/1 -> pqr to eidot/1(pqr)
  Divide/1 -> Quaternion/1, pqr to eidot/2(e0e1e2e3)
  Norme/1(||V||) -> Divide/2
  e0 e1 e2 e3/1 -> Divide/1, Norme/1(V)
  Constant1/1 -> deg2rad/1
  pqr to eidot/1(eidot) -> e0 e1 e2 e3/1
  Euler2Quaternion/1(Quaternion) -> e0 e1 e2 e3/2

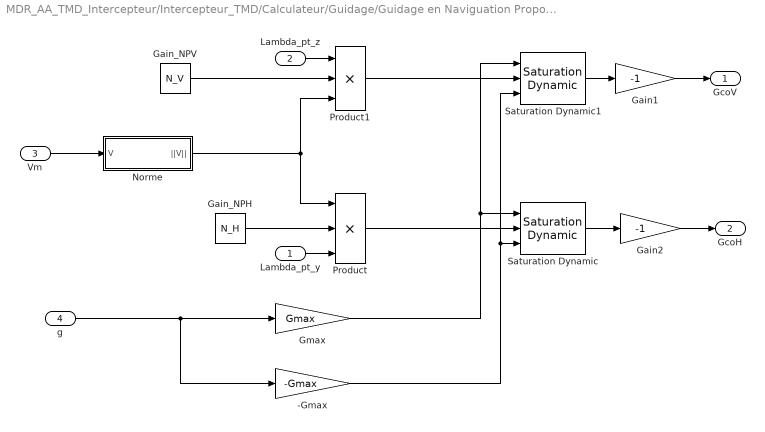
== system MDR_AA_TMD_Intercepteur/Intercepteur_TMD/Calculateur/Guidage/Guidage en Naviguation Proportionnelle 2 axes ==
  Lambda_pt_y : Inport
  Lambda_pt_z : Inport  Port=2
  Vm : Inport  Port=3
  g : Inport  Port=4
  -Gmax : Gain  Gain=-Gmax
  Gain1 : Gain  Gain=-1
  Gain2 : Gain  Gain=-1
  Gain_NPH : Constant  Value=N_H
  Gain_NPV : Constant  Value=N_V
  Gmax : Gain  Gain=Gmax
  Norme : Subsystem  mask(Norme){}
      mask help: Calcul la norme quadratique d'un vecteur.
      mask Help: eval('OpenHelp(''A3_NG.mdl'', ''Help\html\A3_NG_Model_Norme.html'')');
  Product : Product  Inputs=3  RndMeth=Zero
  Product1 : Product  Inputs=3  RndMeth=Zero
  Saturation Dynamic : simulink/Discontinuities/Saturation Dynamic  OutMin=[]  OutMax=[]  OutDataTypeStr=Inherit: Same as second input  OutDataType=fixdt(1, 16)  OutScaling=2^-10  DoSatur=off
  Saturation Dynamic1 : simulink/Discontinuities/Saturation Dynamic  OutMin=[]  OutMax=[]  OutDataTypeStr=Inherit: Same as second input  OutDataType=fixdt(1, 16)  OutScaling=2^-10  DoSatur=off
  GcoV : Outport  PortDimensions=1  VectorParamsAs1DForOutWhenUnconnected=off
  GcoH : Outport  Port=2  PortDimensions=1  VectorParamsAs1DForOutWhenUnconnected=off
  wires:
  Product1/1 -> Saturation Dynamic1/2
  Product/1 -> Saturation Dynamic/2
  Vm/1 -> Norme/1(V)
  Lambda_pt_z/1 -> Product1/1
  Gain_NPV/1 -> Product1/2
  Lambda_pt_y/1 -> Product/3
  Gain_NPH/1 -> Product/2
  Norme/1(||V||) -> Product1/3, Product/1
  Gain1/1 -> GcoV/1
  Gain2/1 -> GcoH/1
  g/1 -> Gmax/1, -Gmax/1
  Gmax/1 -> Saturation Dynamic1/1, Saturation Dynamic/1
  -Gmax/1 -> Saturation Dynamic1/3, Saturation Dynamic/3
  Saturation Dynamic1/1 -> Gain1/1
  Saturation Dynamic/1 -> Gain2/1

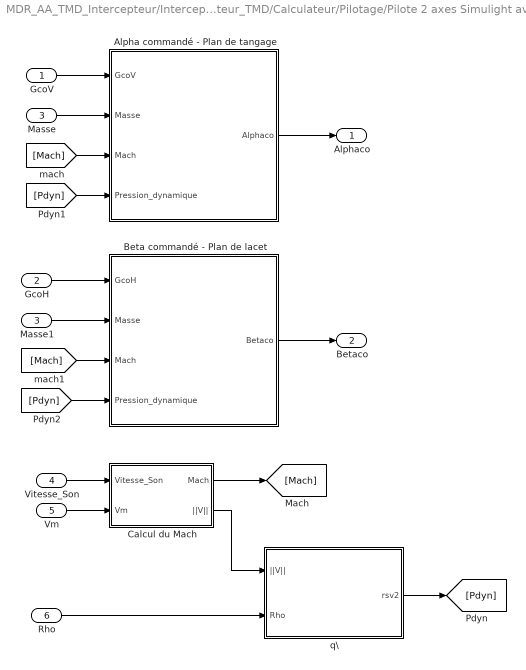
== system MDR_AA_TMD_Intercepteur/Intercepteur_TMD/Calculateur/Pilotage/Pilote 2 axes Simulight avec prise en compte de la manoeuvrabilité max ==
  GcoV : Inport
  GcoH : Inport  Port=2
  Masse : Inport  Port=3
  Vitesse_Son : Inport  Port=4
  Vm : Inport  Port=5
  Rho : Inport  Port=6
  Alpha commandé - Plan de tangage : Subsystem
  Beta commandé - Plan de lacet : Subsystem
  Calcul du Mach : Subsystem
  Masse1 : InportShadow  Port=3
  q\ : Subsystem
  Alphaco : Outport  VectorParamsAs1DForOutWhenUnconnected=off
  Betaco : Outport  Port=2  VectorParamsAs1DForOutWhenUnconnected=off
  wires:
  [Pdyn] -> Beta commandé - Plan de lacet/4(Pression_dynamique)
  [Pdyn] -> Alpha commandé - Plan de tangage/4(Pression_dynamique)
  Rho/1 -> q\/2(Rho)
  Calcul du Mach/2(||V||) -> q\/1(||V||)
  q\/1(rsv2) -> [Pdyn]
  Masse/1 -> Alpha commandé - Plan de tangage/2(Masse)
  Alpha commandé - Plan de tangage/1(Alphaco) -> Alphaco/1
  GcoV/1 -> Alpha commandé - Plan de tangage/1(GcoV)
  GcoH/1 -> Beta commandé - Plan de lacet/1(GcoH)
  Masse1/1 -> Beta commandé - Plan de lacet/2(Masse)
  Beta commandé - Plan de lacet/1(Betaco) -> Betaco/1
  Vitesse_Son/1 -> Calcul du Mach/1(Vitesse_Son)
  Vm/1 -> Calcul du Mach/2(Vm)
  Calcul du Mach/1(Mach) -> [Mach]
  [Mach] -> Alpha commandé - Plan de tangage/3(Mach)
  [Mach] -> Beta commandé - Plan de lacet/3(Mach)

== system MDR_AA_TMD_Intercepteur/Intercepteur_TMD/Forces-Moments/Aerodynamique 3D (CA//CY//CN) v1.0/Plan de lacet ==
  rsv2 : Inport
  Mach : Inport  Port=2
  BetaR : Inport  Port=3
  Calcul de CN0 : Subsystem
  Gain : Gain  Gain=-1
  Product7 : Product  Inputs=**  RndMeth=Zero
  rad2deg : Gain  Gain=180/pi
  Y0 : Outport  VectorParamsAs1DForOutWhenUnconnected=off
  wires:
  Product7/1 -> Gain/1
  Mach/1 -> Calcul de CN0/1(Mach)
  rad2deg/1 -> Calcul de CN0/2(Beta)
  BetaR/1 -> rad2deg/1
  Calcul de CN0/1(CY0) -> Product7/2
  rsv2/1 -> Product7/1
  Gain/1 -> Y0/1

== system MDR_AA_TMD_Intercepteur/Intercepteur_TMD/Forces-Moments/Aerodynamique 3D (CA//CY//CN) v1.0/Plan de tangage ==
  rsv2 : Inport
  Mach : Inport  Port=2
  AlphaR : Inport  Port=3
  Calcul de CN0 : Subsystem
  Gain : Gain  Gain=-1
  Product7 : Product  Inputs=**  RndMeth=Zero
  rad2deg : Gain  Gain=180/pi
  N0 : Outport  VectorParamsAs1DForOutWhenUnconnected=off
  wires:
  Product7/1 -> Gain/1
  Calcul de CN0/1(CN0) -> Product7/2
  rad2deg/1 -> Calcul de CN0/2(Alpha)
  AlphaR/1 -> rad2deg/1
  rsv2/1 -> Product7/1
  Mach/1 -> Calcul de CN0/1(Mach)
  Gain/1 -> N0/1

== system MDR_AA_TMD_Intercepteur/Intercepteur_TMD/Forces-Moments/Aerodynamique 3D (CA//CY//CN) v1.0/Pression Dynamique Mach ==
  Vm : Inport
  Rho : Inport  Port=2
  Vson : Inport  Port=3
  Divide : Product  Inputs=*/
  Norme : Subsystem  mask(Norme){}
      mask help: Calcul la norme quadratique d'un vecteur.
      mask Help: eval('OpenHelp(''A3_NG.mdl'', ''Help\html\A3_NG_Model_Norme.html'')');
  q\ : Subsystem
  rsv2 : Outport  VectorParamsAs1DForOutWhenUnconnected=off
  Mach : Outport  Port=2  VectorParamsAs1DForOutWhenUnconnected=off
  wires:
  Norme/1(||V||) -> q\/2(||V||), Divide/1
  Rho/1 -> q\/1(Rho)
  Vm/1 -> Norme/1(V)
  Vson/1 -> Divide/2
  q\/1(rsv2) -> rsv2/1
  Divide/1 -> Mach/1

== system MDR_AA_TMD_Intercepteur/Intercepteur_TMD/Forces-Moments/Aerodynamique 3D (CA//CY//CN) v1.0/Trainée ==
  rsv2 : Inport
  Mach : Inport  Port=2
  Ok_Propu : Inport  Port=3
  Altitude : Inport  Port=4
  Calcul de CA non propu : Subsystem
  Calcul de CA propu : Subsystem
  Changement de sens pour l'altitude qui est négative dans le modèle NED : Gain  Gain=-1
  Gain : Gain  Gain=-1
  Product : Product  RndMeth=Zero
  Switch : Switch  Criteria=u2 ~= 0
  A0 : Outport  VectorParamsAs1DForOutWhenUnconnected=off
  wires:
  Product/1 -> Gain/1
  Mach/1 -> Calcul de CA propu/1(Mach), Calcul de CA non propu/1(Mach)
  Ok_Propu/1 -> Switch/2
  Calcul de CA propu/1(CA) -> Switch/1
  Calcul de CA non propu/1(CA) -> Switch/3
  Switch/1 -> Product/2
  Altitude/1 -> Changement de sens pour l'altitude qui est négative dans le modèle NED/1
  Changement de sens pour l'altitude qui est négative dans le modèle NED/1 -> Calcul de CA propu/2(Altitude), Calcul de CA non propu/2(Altitude)
  rsv2/1 -> Product/1
  Gain/1 -> A0/1

== system MDR_AA_TMD_Intercepteur/Intercepteur_TMD/Forces-Moments/Aerodynamique 3D (CA//CY//CN) v1.0/Vectorisation ==
  Ax_Aero : Inport
  Ay_Aero : Inport  Port=2
  Az_Aero : Inport  Port=3
  Vector Concatenate : Concatenate  NumInputs=3
  Faero : Outport  VectorParamsAs1DForOutWhenUnconnected=off
  wires:
  Az_Aero/1 -> Vector Concatenate/3
  Ax_Aero/1 -> Vector Concatenate/1
  Ay_Aero/1 -> Vector Concatenate/2
  Vector Concatenate/1 -> Faero/1

== system MDR_AA_TMD_Intercepteur/Intercepteur_TMD/Forces-Moments/Propulsion de l'exemple TMD/Concaténation des deux phases de poussée ==
  Poussee_Boost : Inport
  Poussee_Croisiere : Inport  Port=2
  Debit_Boost : Inport  Port=3
  Debit_Croisiere : Inport  Port=4
  Add : Sum
  Add1 : Sum
  Vectorisation de la poussée : Gain  Gain=[1 0 0]
  Fpropu : Outport
  debit_carburant : Outport  Port=2
  wires:
  Debit_Boost/1 -> Add/2
  Add1/1 -> debit_carburant/1
  Debit_Croisiere/1 -> Add1/2
  Poussee_Croisiere/1 -> Add1/1
  Add/1 -> Vectorisation de la poussée/1
  Poussee_Boost/1 -> Add/1
  Vectorisation de la poussée/1 -> Fpropu/1

== system MDR_AA_TMD_Intercepteur/Intercepteur_TMD/Forces-Moments/Propulsion de l'exemple TMD/Propulsion Booster ==
  Pression_statique : Inport
  Add : Sum  Inputs=+-
  Calcul de la force de poussée : Subsystem
  Calcul du débit de carburant : Subsystem  TreatAsAtomicUnit=on
  Clock : Clock
  Clock1 : Clock
  Clock2 : Clock
  Saturation : Saturate  UpperLimit=Inf  LowerLimit=0
  Switch : Switch  Criteria=u2 > Threshold  Threshold=t_b+Retard_Propu
  Switch1 : Switch  Criteria=u2 > Threshold  Threshold=Retard_Propu
  constant : Constant  Value=0
  constant1 : Constant  Value=Retard_Propu
  constant2 : Constant  Value=0
  constant3 : Constant  Value=g0
  Force_poussee : Outport  VectorParamsAs1DForOutWhenUnconnected=off
  debit_propu : Outport  Port=2  VectorParamsAs1DForOutWhenUnconnected=off
  wires:
  Switch/1 -> debit_propu/1, Calcul de la force de poussée/1(debit_propu)
  constant/1 -> Switch/1
  Clock1/1 -> Switch/2
  Calcul de la force de poussée/1(Force_poussee) -> Force_poussee/1
  constant3/1 -> Calcul de la force de poussée/2(g0)
  Pression_statique/1 -> Calcul de la force de poussée/3(Pression_statique)
  Add/1 -> Saturation/1
  Clock/1 -> Add/1
  constant1/1 -> Add/2
  Saturation/1 -> Calcul du débit de carburant/1(t)
  Calcul du débit de carburant/1(debit_propu) -> Switch1/1
  Clock2/1 -> Switch1/2
  constant2/1 -> Switch1/3
  Switch1/1 -> Switch/3

== system MDR_AA_TMD_Intercepteur/Intercepteur_TMD/Forces-Moments/Propulsion de l'exemple TMD/Propulsion Croisiere ==
  Pression_statique : Inport
  Add : Sum  Inputs=+-
  Calcul de la force de poussée : Subsystem
  Calcul du débit de carburant : Subsystem  TreatAsAtomicUnit=on
  Clock : Clock
  Clock1 : Clock
  Clock2 : Clock
  Saturation : Saturate  UpperLimit=Inf  LowerLimit=0
  Switch : Switch  Criteria=u2 > Threshold  Threshold=t_b+Retard_Propu
  Switch1 : Switch  Criteria=u2 > Threshold  Threshold=Retard_Propu
  constant : Constant  Value=0
  constant1 : Constant  Value=Retard_Propu
  constant2 : Constant  Value=0
  constant3 : Constant  Value=g0
  Force_poussee : Outport  VectorParamsAs1DForOutWhenUnconnected=off
  debit_propu : Outport  Port=2  VectorParamsAs1DForOutWhenUnconnected=off
  wires:
  Switch/1 -> debit_propu/1, Calcul de la force de poussée/1(debit_propu)
  constant/1 -> Switch/1
  Clock1/1 -> Switch/2
  Calcul de la force de poussée/1(Force_poussee) -> Force_poussee/1
  constant3/1 -> Calcul de la force de poussée/2(g0)
  Pression_statique/1 -> Calcul de la force de poussée/3(Pression_statique)
  Add/1 -> Saturation/1
  Clock/1 -> Add/1
  constant1/1 -> Add/2
  Saturation/1 -> Calcul du débit de carburant/1(t)
  Calcul du débit de carburant/1(debit_propu) -> Switch1/1
  Clock2/1 -> Switch1/2
  constant2/1 -> Switch1/3
  Switch1/1 -> Switch/3

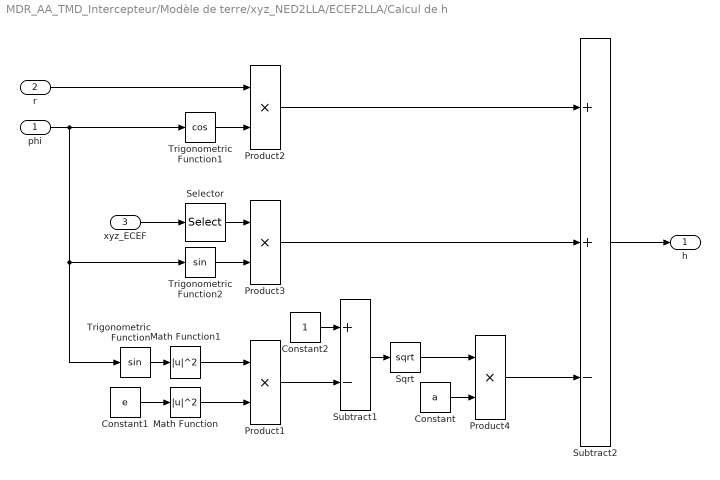
== system MDR_AA_TMD_Intercepteur/Modèle de terre/xyz_NED2LLA/ECEF2LLA/Calcul de h ==
  phi : Inport
  r : Inport  Port=2
  xyz_ECEF : Inport  Port=3
  Constant : Constant  Value=a
  Constant1 : Constant  Value=e
  Constant2 : Constant
  Math Function : Math  Operator=magnitude^2  SaturateOnIntegerOverflow=on
  Math Function1 : Math  Operator=magnitude^2  SaturateOnIntegerOverflow=on
  Product{1..4} (4 alike) : Product
  Selector : Selector  InputPortWidth=3  IndexOptions=Index vector (dialog)  Indices=[3]  OutputSizes=1
  Sqrt : Sqrt  SaturateOnIntegerOverflow=on
  Subtract1 : Sum  Inputs=+-
  Subtract2 : Sum  Inputs=++-
  Trigonometric Function : Trigonometry
  Trigonometric Function1 : Trigonometry  Operator=cos
  Trigonometric Function2 : Trigonometry
  h : Outport  VectorParamsAs1DForOutWhenUnconnected=off
  wires:
  Math Function1/1 -> Product1/1
  Math Function/1 -> Product1/2
  Trigonometric Function/1 -> Math Function1/1
  Constant1/1 -> Math Function/1
  Trigonometric Function1/1 -> Product2/2
  r/1 -> Product2/1
  Trigonometric Function2/1 -> Product3/2
  xyz_ECEF/1 -> Selector/1
  Selector/1 -> Product3/1
  phi/1 -> Trigonometric Function2/1, Trigonometric Function/1, Trigonometric Function1/1
  Product1/1 -> Subtract1/2
  Subtract1/1 -> Sqrt/1
  Constant/1 -> Product4/2
  Constant2/1 -> Subtract1/1
  Sqrt/1 -> Product4/1
  Product2/1 -> Subtract2/1
  Product3/1 -> Subtract2/2
  Product4/1 -> Subtract2/3
  Subtract2/1 -> h/1

== system MDR_AA_TMD_Intercepteur/Modèle de terre/xyz_NED2LLA/ECEF2LLA/Calcul de la latitude ==
  xyz_ECEF : Inport
  r : Inport  Port=2
  Calcul de mu : Subsystem
  Trigonometric Function1 : Trigonometry  Operator=atan2
  den(Phi) : Subsystem
  num(Phi) : Subsystem
  Phi : Outport  VectorParamsAs1DForOutWhenUnconnected=off
  wires:
  r/1 -> den(Phi)/2(r), Calcul de mu/2(r)
  Calcul de mu/1(mu) -> den(Phi)/1(mu), num(Phi)/1(mu)
  xyz_ECEF/1 -> num(Phi)/2(xyz_ECEF), Calcul de mu/1(xyz_ECEF)
  num(Phi)/1(num_phi) -> Trigonometric Function1/1
  den(Phi)/1(den_phi) -> Trigonometric Function1/2
  Trigonometric Function1/1 -> Phi/1

== system MDR_AA_TMD_Intercepteur/Modèle de terre/xyz_NED2LLA/ECEF2LLA/Calcul de la longitude ==
  xyz_ECEF : Inport
  Selector1 : Selector  InputPortWidth=3  IndexOptions=Index vector (dialog)  Indices=[2]  OutputSizes=1
  Selector2 : Selector  InputPortWidth=3  IndexOptions=Index vector (dialog)  Indices=[1]  OutputSizes=1
  Trigonometric Function1 : Trigonometry  Operator=atan2
  Lambda : Outport  VectorParamsAs1DForOutWhenUnconnected=off
  wires:
  Selector1/1 -> Trigonometric Function1/1
  Selector2/1 -> Trigonometric Function1/2
  Trigonometric Function1/1 -> Lambda/1
  xyz_ECEF/1 -> Selector2/1, Selector1/1

== system MDR_AA_TMD_Intercepteur/Modèle de terre/xyz_NED2LLA/ECEF2LLA/Calcul de r ==
  xyz_ECEF : Inport
  Norme : Subsystem  mask(Norme){}
      mask help: Calcul la norme quadratique d'un vecteur.
      mask Help: eval('OpenHelp(''A3_NG.mdl'', ''Help\html\A3_NG_Model_Norme.html'')');
  Selector : Selector  InputPortWidth=3  IndexOptions=Index vector (dialog)  Indices=[1 2]  OutputSizes=1
  r : Outport  VectorParamsAs1DForOutWhenUnconnected=off
  wires:
  Norme/1(||V||) -> r/1
  xyz_ECEF/1 -> Selector/1
  Selector/1 -> Norme/1(V)

== system MDR_AA_TMD_Intercepteur/Modèle de terre/xyz_NED2LLA/xyz_ENU2ECEF/Matrice de passage du repère NED au repère ECEF ==
  Col 1 : Subsystem
  Col 2 : Subsystem
  Col 3 : Subsystem
  Matrix Concatenate : Concatenate  NumInputs=3  Mode=Multidimensional array  ConcatenateDimension=2
  Reshape : Reshape  OutputDimensionality=Column vector (2-D)
  Reshape1 : Reshape  OutputDimensionality=Column vector (2-D)
  Reshape2 : Reshape  OutputDimensionality=Column vector (2-D)
  M_NED2ECEF : Outport  VectorParamsAs1DForOutWhenUnconnected=off
  wires:
  Matrix Concatenate/1 -> M_NED2ECEF/1
  Col 3/1(C3) -> Reshape2/1
  Col 2/1(C2) -> Reshape1/1
  Col 1/1(C1) -> Reshape/1
  Reshape/1 -> Matrix Concatenate/1
  Reshape1/1 -> Matrix Concatenate/2
  Reshape2/1 -> Matrix Concatenate/3
